simulink model "tqdtqr_rebuild_V3"  (R2021b)
settings: Solver=VariableStepAuto  StartTime=0.0  StopTime=10.0  RelTol=1e-3
undefined symbols (not defined in the file): ATQD_AfterTqMinGain_X_Deg, ATQD_APSCreepBaseTqD_X_kph, ATQD_APSCreepBaseTqD_Y_Deg, ATQD_APSCreepBaseTqR_X_kph, ATQD_APSCreepBaseTqR_Y_Deg, ATQD_APSCreepIterm_X_kph, ATQD_APSCreepIterm_Y_kph, ATQD_APSCreepPterm_X_kph, ATQD_APSCreepPterm_Y_kph, ATQD_APSDecReq_X_kph, ATQD_APSDecReq_Y_mps2, ATQD_APSDecReqCMD_X_kph, ATQD_APSDecReqTs_X_pct, ATQD_APSDecTimeGain_X_Deg, ATQD_APSDecTimeGain_Y_s, ATQD_APSReqLowSpd_X_Deg, ATQD_AutoHoldReleaseBPS_X_Deg, ATQD_AWDLoadTrqnsGain_X_kg, ATQD_AWDLoadTrqnsGain_Y_pct, ATQD_BOSEnBPSPosn_X_kph, ATQD_BOSMap_X_rpm, ATQD_BOSMap_Y_pct, ATQD_CreepBaseTqD_X_kph, ATQD_CreepBaseTqD_Y_Deg, ATQD_CreepBaseTqR_X_kph, ATQD_CreepBaseTqR_Y_Deg, ATQD_CreepBPSDisPosn_X_Deg, ATQD_CreepBPSDisPosnR_X_Deg, ATQD_CreepBPSEnPosn_X_Deg, ATQD_CreepBPSEnPosnR_X_Deg, ATQD_CreepDeltaTq_X_kph, ATQD_CreepIterm_X_kph, ATQD_CreepIterm_Y_kph, ATQD_CreepItermMaxLimit_X_pct, ATQD_CreepPreloadTime_X_kph, ATQD_CreepPreloadTq_X_kph, ATQD_CreepPreloadTq_Y_s, ATQD_CreepProtTq_X_Deg, ATQD_CreepPterm_X_kph, ATQD_CreepPterm_Y_kph, ATQD_CreepRrTqSpRat_X_rpm, ATQD_CreepRrTqSpRat_Y_Nm, ATQD_CreepTargetSpdD_X_pct, ATQD_CreepTargetSpdR_X_pct, ATQD_CreepUpLimitTq_X_rpm, ATQD_DecIneOPDHoldEnDelay_X_Deg, ATQD_DecIneOPDHoldEnDelay_Y_bar, ATQD_ECOTqMapD_X_rpm, ATQD_ECOTqMapD_Y_pct, ATQD_EMTqMapD_X_rpm, ATQD_EMTqMapD_Y_pct, ATQD_EOPDTqMapDCon_X_rpm, ATQD_EOPDTqMapDCon_Y_Deg, ATQD_EstInitVehWeight_X_c, ATQD_FAfterTqCMDGain_X_rpm, ATQD_FAfterTqCMDGain_Y_pct, ATQD_ForceLowSpd_X_Deg, ATQD_ForcePLimitSpd_X_Deg, ATQD_FrLossMAPLowV_X_rpm, ATQD_FrLossMAPLowV_Y_Nm ... (+949)
libraries: simulink x235, hcu_lib x208, tqr x63, tqd x6
(part 13 of 37)

== system tqdtqr_rebuild_V3/Input_Convert/Signal function/SWC1 SWC2 status ==
  note: SWC1 SWC2 result merge
  note: SWC2 status
  note: SWC1 status
  BSCPIn_outputs : Inport
  BSignalConvert_outputs : Inport  Port=2
  VTQD_GearActualPosn_enum : Inport  Port=3
  Bus Selector : BusSelector  OutputSignals=task_time_s,VINP_SWCResUpSta_flg,VINP_SWCSetdownSta_flg,VINP_SWCACCSta_flg,VINP_SWCCANCELSta_flg,VINP_IVIISAOffsetSpd_enum,VINP_ADASISASta_enum,VPMM_PowerSta_enum,VINP_ADASACCSta_enum,VVMC_CCCtrlSta_enum,VVMC_MSACtrlSta_enum,VINP_ADASVehSpdLim_enum,VVMC_LVDAACCStatusInformation_flg,VVMC_ACCObjDist_m,VVMC_MeterIndSpeed_raw32,VINP_Distanceunit_flg,VINP_SmartEcoModeSW_flg,VVMC_SetACCDisableAPS_flg,VINP_SWC2LScrollUpSta_flg,VINP_SWC2LScrollDownSta_flg,VINP_SWC2LScrollPressSta_flg,VINP_SWC2LADASSta_flg,VVMC_ADASActive_flg,VVMC_MSAActive_flg,VINP_ADASSLIFSpdLim_enum,VINP_IVIACCAdaptiveSta_flg,VTQD_LowIdleAccPedal_flg,VINP_SWCType_enum
  Bus Selector1 : BusSelector  OutputSignals=VTQD_ShiftGearPosn_enum
  Constant{1..3,90} (4 alike) : Constant  Value=ENUM_SWCTYPE_SWC2
  Constant77 : Constant  Value=ENUM_SWCTYPE_SWC
  Constant{78,82,84,89} (4 alike) : Constant  Value=FALSE
  Data Type Conversion4 : DataTypeConversion  OutDataTypeStr=boolean
  Data Type Conversion5 : DataTypeConversion  OutDataTypeStr=boolean
  Equal{1..3,30,40} (5 alike) : RelationalOperator  Operator===  OutDataTypeStr=boolean  RndMeth=Simplest
  SWC2_Subsystem : Subsystem  TreatAsAtomicUnit=on
  SWC_Subsystem : Subsystem
  Switch : Switch  Criteria=u2 ~= 0
      settings: AttributesFormatString=%<Criteria>
  Switch1 : Switch  Criteria=u2 ~= 0
      settings: AttributesFormatString=%<Criteria>
  Switch2 : Switch  Criteria=u2 ~= 0
      settings: AttributesFormatString=%<Criteria>
  VTQD_SWCResUpSta_flg : Outport
  VTQD_SWCSetdownSta_flg : Outport  Port=2
  VTQD_SWCCancelSta_flg : Outport  Port=3
  VTQD_SpdCtrlMode_enum : Outport  Port=4
  VTQD_SpdCtrlSta_flg : Outport  Port=5
  VTQD_SetSpd_kph : Outport  Port=6
  VTQD_SWC2ResUpSta_flg : Outport  Port=7
  VTQD_SWC2SetdownSta_flg : Outport  Port=8
  VTQD_SWC2CancelSta_flg : Outport  Port=9
  VTQD_SWC2LADASSta_flg : Outport  Port=10
  VTQD_SpdLim4SetSpd_raw32 : Outport  Port=11
  VTQD_SWC2ScrollUpSta_flg : Outport  Port=12
  VTQD_SWC1SetSpd_kph : Outport  Port=13
  VTQD_SWC2SetSpd_kph : Outport  Port=14
  wires:
  [VVMC_CCCtrlSta_enum] -> SWC_Subsystem/14(VVMC_CCCtrlSta_enum)
  [VINP_ADASACCSta_enum] -> SWC_Subsystem/11(VINP_ADASACCSta_enum)
  [VPMM_PowerSta_enum] -> SWC_Subsystem/10(VPMM_PowerSta_enum)
  [VINP_SWCACCSta_flg] -> SWC_Subsystem/6(VINP_SWCACCSta_flg)
  [VINP_SWCCANCELSta_flg] -> SWC_Subsystem/8(VINP_SWCCANCELSta_flg)
  [VINP_IVIISAOffsetSpd_enum] -> SWC_Subsystem/9(VTQD_IVIISAOffsetSpd_enum)
  [VINP_ADASVehSpdLim_enum] -> SWC_Subsystem/16(VINP_ADASVehSpdLim_kph)
  [VVMC_ACCObjDist_m] -> SWC_Subsystem/19(VVMC_ACCObjDist_m)
  [VDDM_SWCACCSta_flg] -> SWC_Subsystem/5(VDDM_SWCACCSta_flg)
  SWC_Subsystem/4(VTQD_SWCSpdCtrlMode_enum) -> [VTQD_SWCSpdCtrlMode_enum]
  SWC_Subsystem/2(VTQD_SWCSetdownSta_flg) -> [VTQD_SWCSetdownSta_flg]
  [VDDM_SWCCANCELSta_flg] -> SWC_Subsystem/7(VDDM_SWCCANCELSta_flg)
  Constant77/1 -> Equal30/2
  SWC_Subsystem/1(VTQD_SWCResUpSta_flg) -> [VTQD_SWCResUpSta_flg]
  [VDDM_SWCResUpSta_flg] -> SWC_Subsystem/1(VDDM_SWCResUpSta_flg)
  SWC_Subsystem/5(VTQD_SWCSpdCtrlSta_flg) -> [VTQD_SWCSpdCtrlSta_flg]
  Equal30/1 -> Data Type Conversion4/1
  Constant78/1 -> [VDDM_SWCResUpSta_flg]  "VDDM_SWCRegenUpSta_flg"
  SWC_Subsystem/6(VTQD_SWC1SetSpd_kph) -> [VTQD_SWC1SetSpd_kph]
  [VVMC_MeterIndSpeed_raw32] -> SWC_Subsystem/20(VVMC_MeterIndSpeed_raw32)
  [VINP_ADASISASta_enum] -> SWC_Subsystem/12(VINP_ADASISASta_enum)
  Constant82/1 -> [VDDM_SWCSetdownSta_flg]  "VDDM_SWCRegenDownSta_flg"
  Constant84/1 -> [VDDM_SWCACCSta_flg]  "VDDM_SWCRegenDownSta_flg"
  [VINP_SWCResUpSta_flg] -> SWC_Subsystem/2(VINP_SWCResUpSta_flg)
  Data Type Conversion4/1 -> SWC_Subsystem/Enable
  [VDDM_SWCSetdownSta_flg] -> SWC_Subsystem/3(VDDM_SWCSetdownSta_flg)
  [VTQD_ShiftGearPosn_enum] -> SWC_Subsystem/13(VTQD_ShiftGearPosn_enum)
  [VVMC_LVDAACCStatusInformation_flg] -> SWC_Subsystem/18(VVMC_LVDAACCStatusInformation_flg)
  [VINP_SWCSetdownSta_flg] -> SWC_Subsystem/4(VINP_SWCSetdownSta_flg)
  Constant89/1 -> [VDDM_SWCCANCELSta_flg]  "VDDM_SWCRegenDownSta_flg"
  [task_time_s] -> SWC_Subsystem/17(task_time_s)
  [VVMC_SetACCDisableAPS_flg] -> SWC_Subsystem/23(VVMC_SetACCDisableAPS_flg)
  [VINP_Distanceunit_flg] -> SWC_Subsystem/21(VINP_Distanceunit_flg)
  [VINP_SmartEcoModeSW_flg] -> SWC_Subsystem/22(VINP_SmartEcoModeSW_flg)
  [VVMC_MSACtrlSta_enum] -> SWC_Subsystem/15(VVMC_MSACtrlSta_enum)
  [VINP_SWCType_enum] -> Equal30/1
  SWC_Subsystem/3(VTQD_SWCCancelSta_flg) -> [VTQD_SWCCancelSta_flg]
  BSCPIn_outputs/1 -> Bus Selector/1
  Bus Selector/2 -> [VINP_SWCResUpSta_flg]  "<VINP_SWCResUpSta_flg>"
  Bus Selector/3 -> [VINP_SWCSetdownSta_flg]  "<VINP_SWCSetdownSta_flg>"
  Bus Selector/4 -> [VINP_SWCACCSta_flg]  "<VINP_SWCACCSta_flg>"
  Bus Selector/5 -> [VINP_SWCCANCELSta_flg]  "<VINP_SWCCANCELSta_flg>"
  Bus Selector/6 -> [VINP_IVIISAOffsetSpd_enum]  "<VINP_IVIISAOffsetSpd_enum>"
  Bus Selector/7 -> [VINP_ADASISASta_enum]  "<VINP_ADASISASta_enum>"
  Bus Selector/8 -> [VPMM_PowerSta_enum]  "<VPMM_PowerSta_enum>"
  Bus Selector/9 -> [VINP_ADASACCSta_enum]  "<VINP_ADASACCSta_enum>"
  Bus Selector/1 -> [task_time_s]  "<task_time_s>"
  Bus Selector/15 -> [VVMC_MeterIndSpeed_raw32]  "<VVMC_MeterIndSpeed_raw32>"
  Bus Selector/17 -> [VINP_SmartEcoModeSW_flg]  "<VINP_SmartEcoModeSW_flg>"
  Bus Selector/18 -> [VVMC_SetACCDisableAPS_flg]  "<VVMC_SetACCDisableAPS_flg>"
  Bus Selector/19 -> [VINP_SWC2LScrollUpSta_flg]  "<VINP_SWC2LScrollUpSta_flg>"
  Bus Selector/20 -> [VINP_SWC2LScrollDownSta_flg]  "<VINP_SWC2LScrollDownSta_flg>"
  Bus Selector/24 -> [VVMC_MSAActive_flg]  "<VVMC_MSAActive_flg>"
  Bus Selector/26 -> [VINP_IVIACCAdaptiveSta_flg]  "<VINP_IVIACCAdaptiveSta_flg>"
  Bus Selector/25 -> [VINP_ADASSLIFSpdLim_enum]  "<VINP_ADASSLIFSpdLim_enum>"
  Bus Selector/27 -> [VTQD_LowIdleAccPedal_flg]  "<VTQD_LowIdleAccPedal_flg>"
  VTQD_GearActualPosn_enum/1 -> [VTQD_GearActualPosn_enum]
  BSignalConvert_outputs/1 -> Bus Selector1/1
  Bus Selector1/1 -> [VTQD_ShiftGearPosn_enum]  "<VTQD_ShiftGearPosn_enum>"
  Bus Selector/28 -> [VINP_SWCType_enum]  "<VINP_SWCType_enum>"
  Bus Selector/10 -> [VVMC_CCCtrlSta_enum]  "<VVMC_CCCtrlSta_enum>"
  Bus Selector/11 -> [VVMC_MSACtrlSta_enum]  "<VVMC_MSACtrlSta_enum>"
  Bus Selector/12 -> [VINP_ADASVehSpdLim_enum]  "<VINP_ADASVehSpdLim_enum>"
  Bus Selector/13 -> [VVMC_LVDAACCStatusInformation_flg]  "<VVMC_LVDAACCStatusInformation_flg>"
  Bus Selector/14 -> [VVMC_ACCObjDist_m]  "<VVMC_ACCObjDist_m>"
  Bus Selector/16 -> [VINP_Distanceunit_flg]  "<VINP_Distanceunit_flg>"
  Bus Selector/21 -> [VINP_SWC2LScrollPressSta_flg]  "<VINP_SWC2LScrollPressSta_flg>"
  Bus Selector/22 -> [VINP_SWC2LADASSta_flg]  "<VINP_SWC2LADASSta_flg>"
  Bus Selector/23 -> [VVMC_ADASActive_flg]  "<VVMC_ADASActive_flg>"
  [VINP_SWC2LScrollUpSta_flg] -> SWC2_Subsystem/1(VINP_SWC2LScrollUpSta_flg)
  Data Type Conversion5/1 -> SWC2_Subsystem/Enable
  [VINP_SWC2LScrollDownSta_flg] -> SWC2_Subsystem/2(VINP_SWC2LScrollDownSta_flg)
  [VINP_Distanceunit_flg] -> SWC2_Subsystem/17(VINP_Distanceunit_flg)
  Equal40/1 -> Data Type Conversion5/1
  Constant90/1 -> Equal40/2
  [VVMC_MSAActive_flg] -> SWC2_Subsystem/8(VVMC_MSAActive_flg)
  [VVMC_CCCtrlSta_enum] -> SWC2_Subsystem/19(VVMC_CCCtrlSta_enum)
  SWC2_Subsystem/2(VTQD_SWC2SetdownSta_flg) -> [VTQD_SWC2SetdownSta_flg]
  [VINP_SWC2LADASSta_flg] -> SWC2_Subsystem/4(VINP_SWC2LADASSta_flg)
  [VTQD_GearActualPosn_enum] -> SWC2_Subsystem/5(VTQD_GearActualPosn_enum)
  [VTQD_ShiftGearPosn_enum] -> SWC2_Subsystem/15(VTQD_ShiftGearPosn_enum)
  [VPMM_PowerSta_enum] -> SWC2_Subsystem/14(VPMM_PowerSta_enum)
  [VINP_ADASACCSta_enum] -> SWC2_Subsystem/9(VINP_ADASACCSta_enum)
  SWC2_Subsystem/4(VTQD_SWC2LADASSta_flg) -> [VTQD_SWC2LADASSta_flg]
  [VINP_SWC2LScrollPressSta_flg] -> SWC2_Subsystem/3(VINP_SWC2LScrollPressSta_flg)
  [VINP_IVIACCAdaptiveSta_flg] -> SWC2_Subsystem/18(VINP_IVIACCAdaptiveSta_flg)
  SWC2_Subsystem/3(VTQD_SWC2CancelSta_flg) -> [VTQD_SWC2CancelSta_flg]  "VTQD_SWC2CancelSta_flg"
  [VVMC_ADASActive_flg] -> SWC2_Subsystem/6(VVMC_ADASActive_flg)
  [task_time_s] -> SWC2_Subsystem/12(task_time_s)
  [VINP_SmartEcoModeSW_flg] -> SWC2_Subsystem/20(VINP_SmartEcoModeSW_flg)
  [VINP_IVIISAOffsetSpd_enum] -> SWC2_Subsystem/13(VINP_IVIISAOffsetSpd_enum)
  SWC2_Subsystem/1(VTQD_SWC2ResUpSta_flg) -> [VTQD_SWC2ResUpSta_flg]
  [VVMC_MSACtrlSta_enum] -> SWC2_Subsystem/16(VVMC_MSACtrlSta_enum)
  [VINP_ADASSLIFSpdLim_enum] -> SWC2_Subsystem/11(VINP_ADASSLIFSpdLim_enum)
  SWC2_Subsystem/7(VTQD_SWC2SpdCtrlSta_flg) -> [VTQD_SWC2SpdCtrlSta_flg]
  [VINP_SWCType_enum] -> Equal40/1
  SWC2_Subsystem/6(VTQD_SpdCtrlMode_enum) -> [VTQD_SWC2SpdCtrlMode_enum]
  SWC2_Subsystem/5(VTQD_SpdLim4SetSpd_raw32) -> [VTQD_SpdLim4SetSpd_raw32]
  [VVMC_MeterIndSpeed_raw32] -> SWC2_Subsystem/10(VVMC_MeterIndSpeed_raw32)
  [VVMC_LVDAACCStatusInformation_flg] -> SWC2_Subsystem/7(VVMC_LVDAACCStaInfor_flg)
  [VTQD_LowIdleAccPedal_flg] -> SWC2_Subsystem/21(VTQD_LowIdleAccPedal_flg)
  [VTQD_SWCResUpSta_flg] -> VTQD_SWCResUpSta_flg/1
  [VTQD_SWCSetdownSta_flg] -> VTQD_SWCSetdownSta_flg/1
  [VTQD_SWCCancelSta_flg] -> VTQD_SWCCancelSta_flg/1
  [VTQD_SpdCtrlMode_enum] -> VTQD_SpdCtrlMode_enum/1
  [VTQD_SetSpd_kph] -> VTQD_SetSpd_kph/1
  [VTQD_SWC2ResUpSta_flg] -> VTQD_SWC2ResUpSta_flg/1
  [VTQD_SWC2SetdownSta_flg] -> VTQD_SWC2SetdownSta_flg/1
  [VTQD_SWC2CancelSta_flg] -> VTQD_SWC2CancelSta_flg/1
  [VTQD_SWC2LADASSta_flg] -> VTQD_SWC2LADASSta_flg/1
  [VTQD_SpdLim4SetSpd_raw32] -> VTQD_SpdLim4SetSpd_raw32/1
  SWC2_Subsystem/9(VTQD_SWC2ScrollUpSta_flg) -> [VTQD_SWC2ScrollUpSta_flg]
  [VTQD_SWC2ScrollUpSta_flg] -> VTQD_SWC2ScrollUpSta_flg/1
  [VTQD_SpdCtrlSta_flg] -> VTQD_SpdCtrlSta_flg/1
  SWC2_Subsystem/8(VTQD_SWC2SetSpd_kph) -> [VTQD_SWC2SetSpd_kph]
  [VINP_SWCType_enum] -> Equal1/1
  Constant1/1 -> Equal1/2
  Equal1/1 -> Switch/2
  [VTQD_SWC1SetSpd_kph] -> Switch/1
  [VTQD_SWC2SetSpd_kph] -> Switch/3
  Switch/1 -> [VTQD_SetSpd_kph]  "VTQD_SetSpd_kph"
  [VTQD_SWC1SetSpd_kph] -> VTQD_SWC1SetSpd_kph/1
  [VTQD_SWC2SetSpd_kph] -> VTQD_SWC2SetSpd_kph/1
  [VINP_SWCType_enum] -> Equal2/1
  Equal2/1 -> Switch1/2
  Constant2/1 -> Equal2/2
  Switch1/1 -> [VTQD_SpdCtrlMode_enum]  "VTQD_SpdCtrlMode_enum"
  [VTQD_SWC2SpdCtrlMode_enum] -> Switch1/3
  [VTQD_SWCSpdCtrlMode_enum] -> Switch1/1
  [VINP_SWCType_enum] -> Equal3/1
  Equal3/1 -> Switch2/2
  Constant3/1 -> Equal3/2
  [VTQD_SWC2SpdCtrlSta_flg] -> Switch2/3
  [VTQD_SWCSpdCtrlSta_flg] -> Switch2/1
  Switch2/1 -> [VTQD_SpdCtrlSta_flg]  "VTQD_SpdCtrlSta_flg"

== system tqdtqr_rebuild_V3/Input_Convert/Signal function/ShiftModule ==
  BSCPIn_outputs : Inport
  BSignalConvert_outputs : Inport  Port=2
  VTQD_EPBCarWashMode_flg : Inport  Port=3
  SWC_RegenUp : Inport  Port=4
  SWC_RegenDown : Inport  Port=5
  DriverWhlTqDemFunc_outputs : Inport  Port=6
  BMain_outputs : Inport  Port=7
  VTQD_OPDHoldAllowPark_flg : Inport  Port=8
  Bus Selector : BusSelector  OutputSignals=task_time_s,VPMM_PowerSta_enum,VINP_DrDoorSW_flg,VVMC_APSShiftPosnReq_enum,VVMC_APSActive_flg,VINP_DriverSeatBeltCmd_flg,VINP_ChrgPlugSta_enum,VINP_DOASta_flg,VINP_CAASSta_enum,VDDM_VCURAPSErrLv2_flg,VDDM_VCURAPSErrLv3_flg,VINP_APSStaSystem_enum,VDDM_Shifter1Err_flg,VDDM_ShifterSigErrCFS_flg,VTQD_ShifterHandleCmd_enum,VTQD_ShifterFailsta_enum,VINP_VehSpeed_kph,VINP_EPBSta_enum,VVMC_EstSlope_Deg,VPMM_DrSeatSta_enum,VTQD_ShifterHandleCmd_enum
  Bus Selector1 : BusSelector  OutputSignals=VTQD_BrkSwSta_flg,VTQD_VehActSpd_kph,VTQD_TMRotateDirction_enum,VTQD_IVIPwrLock_flg,VTQD_FrShaftSpd_rpm,VTQD_RrShaftSpd_rpm
  Bus Selector2 : BusSelector  OutputSignals=VTQD_IVIRockModeEn_flg
  Bus Selector3 : BusSelector  OutputSignals=VTQD_AfterAvailableTqDemFr_Nm,VTQD_AfterAvailableTqDemRr_Nm,VTQR_NoABSFEDUWhlTqReq_Nm,VTQR_NoABSREDUWhlTqReq_Nm
  Constant6 : Constant  Value=ENUM_GEARACTUALPOSN_P
  Constant7 : Constant  Value=ENUM_GEARACTUALPOSN_P
  Data Type Conversion1 : DataTypeConversion
  Data Type Conversion2 : DataTypeConversion
  Data Type Conversion3 : DataTypeConversion  OutDataTypeStr=uint8
  Data Type Conversion4 : DataTypeConversion  OutDataTypeStr=boolean
  Determin Gear State Configuration : Subsystem
  Determine_Actual_Gear_Position : Stateflow chart  TreatAsAtomicUnit=on
  Equal : RelationalOperator  Operator===  OutDataTypeStr=boolean  RndMeth=Simplest
  Equal1 : RelationalOperator  Operator=~=  OutDataTypeStr=boolean  RndMeth=Simplest
  Gear Shift Posn Cmd : Subsystem  Description=GearPosition
  SR_Latch : hcu_lib/Basic_Blocks/SR_Latch
  SR_Latch1 : Subsystem  mask(SR_Latch){}
      mask help: SR latch function.
  VTQD_GearActualPosn_enum : Outport
  VTQD_ParkRequest_flg : Outport  Port=2
  VTQD_PBWLockTO_flg : Outport  Port=3
  VTQD_PBWUnlockTO_flg : Outport  Port=4
  VTQD_DriveProtRemove_flg : Outport  Port=5
  VTQD_DriveProtEn_flg : Outport  Port=6
  VTQD_ForceP_flg : Outport  Port=7
  VTQD_DOALatchReq_flg : Outport  Port=8
  VTQD_ForcePLimitSpd_kph : Outport  Port=9
  wires:
  BSCPIn_outputs/1 -> Bus Selector/1
  Bus Selector/1 -> [task_time_s]  "<task_time_s>"
  Bus Selector/2 -> [VPMM_PowerSta_enum]  "<VPMM_PowerSta_enum>"
  Bus Selector/3 -> [VINP_DrDoorSW_flg]  "<VINP_DrDoorSW_flg>"
  Bus Selector/4 -> [VVMC_APSShiftPosnReq_enum]  "<VVMC_APSShiftPosnReq_enum>"
  Bus Selector/5 -> [VVMC_APSActive_flg]  "<VVMC_APSActive_flg>"
  Bus Selector/6 -> [VINP_DriverSeatBeltCmd_flg]  "<VINP_DriverSeatBeltCmd_flg>"
  Bus Selector/7 -> [VINP_ChrgPlugSta_enum]  "<VINP_ChrgPlugSta_enum>"
  Bus Selector/8 -> [VINP_DOASta_flg]  "<VINP_DOASta_flg>"
  Bus Selector/9 -> [VINP_CAASSta_enum]  "<VINP_CAASSta_enum>"
  Bus Selector/10 -> [VDDM_VCURAPSErrLv2_flg]  "<VDDM_VCURAPSErrLv2_flg>"
  Bus Selector/14 -> [VDDM_ShifterSigErrCFS_flg]  "<VDDM_ShifterSigErrCFS_flg>"
  Bus Selector/13 -> [VDDM_Shifter1Err_flg]  "<VDDM_Shifter1Err_flg>"
  Bus Selector/12 -> [VINP_APSStaSystem_enum]  "<VINP_APSStaSystem_enum>"
  Bus Selector/11 -> [VDDM_VCURAPSErrLv3_flg]  "<VDDM_VCURAPSErrLv3_flg>"
  BSignalConvert_outputs/1 -> Bus Selector1/1
  Bus Selector1/1 -> [VTQD_BrkSwSta_flg]  "<VTQD_BrkSwSta_flg>"
  Bus Selector1/3 -> [VTQD_TMRotateDirction_enum]  "<VTQD_TMRotateDirction_enum>"
  Bus Selector1/4 -> [VTQD_IVIPwrLock_flg]  "<VTQD_IVIPwrLock_flg>"
  Bus Selector1/5 -> [VTQD_FrShaftSpd_rpm]  "<VTQD_FrShaftSpd_rpm>"
  Bus Selector1/6 -> [VTQD_RrShaftSpd_rpm]  "<VTQD_RrShaftSpd_rpm>"
  [VTQD_GearActualPosn_enum] -> VTQD_GearActualPosn_enum/1
  [VTQD_DriveProtRemove_flg] -> VTQD_DriveProtRemove_flg/1
  [VTQD_DriveProtEn_flg] -> VTQD_DriveProtEn_flg/1
  [VTQD_ForceP_flg] -> VTQD_ForceP_flg/1
  [VTQD_PBWUnlockTO_flg] -> VTQD_PBWUnlockTO_flg/1
  [VTQD_PBWLockTO_flg] -> VTQD_PBWLockTO_flg/1
  [VTQD_ParkRequest_flg] -> VTQD_ParkRequest_flg/1
  SWC_RegenDown/1 -> [SWC_RegenDown]
  SWC_RegenUp/1 -> [SWC_RegenUp]
  VTQD_EPBCarWashMode_flg/1 -> [VTQD_EPBCarWashMode_flg]
  Bus Selector/15 -> [VTQD_ShifterHandleCmd_enum]  "<VTQD_ShifterHandleCmd_enum>"
  Bus Selector/16 -> [VTQD_ShifterFailsta_enum]  "<VTQD_ShifterFailsta_enum>"
  Determine_Actual_Gear_Position/3(VTQD_PBWUnlockTO_flg) -> Data Type Conversion2/1
  Data Type Conversion2/1 -> SR_Latch1/1(set)
  Data Type Conversion3/1 -> [VTQD_GearActualPosn_enum]  "VTQD_GearActualPosn_enum"
  Constant7/1 -> Equal1/2
  Determine_Actual_Gear_Position/4(VTQD_ParkRequest_flg) -> Data Type Conversion4/1
  [VTQD_GearActualPosn_enum] -> Equal1/1
  [VTQD_ShifterHandleCmd_enum] -> Gear Shift Posn Cmd/1(VTQD_ShifterHandleCmd_enum)
  [VINP_DriverSeatBeltCmd_flg] -> Gear Shift Posn Cmd/6(VINP_DriverSeatBeltCmd_flg)
  Gear Shift Posn Cmd/3(VTQD_PwrStaAllowDR_flg) -> [VTQD_PwrStaAllowDR_flg]
  Gear Shift Posn Cmd/2(VTQD_PwrStaAllowPN_flg) -> [VTQD_PwrStaAllowPN_flg]
  [VINP_APSStaSystem_enum] -> Gear Shift Posn Cmd/23(VINP_APSStaSystem_enum)
  Constant6/1 -> Equal/2
  Equal/1 -> SR_Latch/2
  [VTQD_OPDHoldAllowPark_flg] -> Gear Shift Posn Cmd/19(VTQD_OPDHoldAllowPark_flg)
  [VTQD_ShifterFailsta_enum] -> Gear Shift Posn Cmd/28(VTQD_ShifterFailsta_enum)
  SR_Latch1/1(latched) -> [VTQD_PBWUnlockTO_flg]  "VTQD_PBWUnlockTO_flg"
  [VDDM_Shifter1Err_flg] -> Gear Shift Posn Cmd/24(VDDM_Shifter1Err_flg)
  [VDDM_VCURAPSErrLv3_flg] -> Gear Shift Posn Cmd/22(VDDM_VCURAPSErrLv3_flg)
  [VTQD_GearActualPosn_enum] -> Equal/1
  [VPMM_PowerSta_enum] -> Gear Shift Posn Cmd/2(VPMM_PowerSta_enum)
  [VTQD_AfterAvailableTqDemFr_Nm] -> Gear Shift Posn Cmd/11(VTQD_AfterAvailableTqDemFr_Nm)
  [SWC_RegenDown] -> Gear Shift Posn Cmd/26(SWC_RegenDown)
  Determine_Actual_Gear_Position/1(VTQD_GearActualPosn_enum) -> Data Type Conversion3/1
  Data Type Conversion4/1 -> [VTQD_ParkRequest_flg]  "VTQD_ParkRequest_flg"
  [task_time_s] -> Gear Shift Posn Cmd/15(task_time_s)
  [VINP_DrDoorSW_flg] -> Gear Shift Posn Cmd/3(VINP_DrDoorSW_flg)
  Data Type Conversion1/1 -> SR_Latch/1
  [VINP_CAASSta_enum] -> Gear Shift Posn Cmd/20(VINP_CAASSta_enum)
  [VDDM_VCURAPSErrLv2_flg] -> Gear Shift Posn Cmd/21(VDDM_VCURAPSErrLv2_flg)
  [VTQD_BrkSwSta_flg] -> Gear Shift Posn Cmd/18(VTQD_BrkSwSta_flg)
  [VTQD_EPBCarWashMode_flg] -> Gear Shift Posn Cmd/7(VTQD_EPBCarWashMode_flg)
  [VINP_DOASta_flg] -> Gear Shift Posn Cmd/16(VINP_DOASta_flg)
  [VTQD_IVIPwrLock_flg] -> Gear Shift Posn Cmd/17(VTQD_IVIPwrLock_flg)
  Gear Shift Posn Cmd/1(VTQD_GearShiftCMD_enum) -> [VTQD_GearShiftCMD_enum]
  Gear Shift Posn Cmd/6(VTQD_ForceP_flg) -> [VTQD_ForceP_flg]
  [VINP_ChrgPlugSta_enum] -> Gear Shift Posn Cmd/9(VINP_ChrgPlugSta_enum)
  [VTQR_NoABSREDUWhlTqReq_Nm] -> Gear Shift Posn Cmd/14(VTQR_NoABSREDUWhlTqReq_Nm)
  Determine_Actual_Gear_Position/2(VTQD_PBWLockTO_flg) -> Data Type Conversion1/1
  [VDDM_ShifterSigErrCFS_flg] -> Gear Shift Posn Cmd/27(VDDM_ShifterSigErrCFS_flg)
  [VTQD_AfterAvailableTqDemRr_Nm] -> Gear Shift Posn Cmd/12(VTQD_AfterAvailableTqDemRr_Nm)
  Equal1/1 -> SR_Latch1/2(reset)
  [VVMC_APSShiftPosnReq_enum] -> Gear Shift Posn Cmd/4(VVMC_APSShiftPosnReq_enum)
  [VTQD_GearActualPosn_enum] -> Gear Shift Posn Cmd/10(VTQD_GearActualPosn_enum)
  [VTQR_NoABSFEDUWhlTqReq_Nm] -> Gear Shift Posn Cmd/13(VTQR_NoABSFEDUWhlTqReq_Nm)
  [VVMC_APSActive_flg] -> Gear Shift Posn Cmd/5(VVMC_APSActive_flg)
  [SWC_RegenUp] -> Gear Shift Posn Cmd/25(SWC_RegenUp)
  Gear Shift Posn Cmd/4(VTQD_DriveProtRemove_flg) -> [VTQD_DriveProtRemove_flg]
  Gear Shift Posn Cmd/5(VTQD_DriveProtEn_flg) -> [VTQD_DriveProtEn_flg]
  SR_Latch/1 -> [VTQD_PBWLockTO_flg]  "VTQD_PBWLockTO_flg"
  [VTQD_BrkSwSta_flg] -> Determin Gear State Configuration/1(VTQD_BrkSwSta_flg)
  [VTQD_GearShiftCMD_enum] -> Determin Gear State Configuration/2(VTQD_GearShiftCMD_enum)
  [VINP_VehSpeed_kph] -> Determin Gear State Configuration/3(VINP_VehSpeed_kph)
  [VTQD_PwrStaAllowDR_flg] -> Determin Gear State Configuration/4(VTQD_PwrStaAllowDR_flg)
  [VTQD_PwrStaAllowPN_flg] -> Determin Gear State Configuration/5(VTQD_PwrStaAllowPN_flg)
  [VTQD_TMRotateDirction_enum] -> Determin Gear State Configuration/6(VTQD_TMRotateDirction_enum)
  [VTQD_EPBCarWashMode_flg] -> Determin Gear State Configuration/7(VTQD_EPBCarWashMode_flg)
  [VVMC_APSActive_flg] -> Determin Gear State Configuration/8(VVMC_APSActive_flg)
  [VTQD_ForceP_flg] -> Determin Gear State Configuration/9(VTQD_ForceP_flg)
  [VTQD_IVIRockModeEn_flg] -> Determin Gear State Configuration/10(VTQD_IVIRockModeEn_flg)
  [VTQD_MaxShaftSpd_rpm] -> Determin Gear State Configuration/11(VTQD_MaxShaftSpd_rpm)
  Determin Gear State Configuration/1(VTQD_GearP2N_flg) -> [VTQD_GearP2N_flg]
  Determin Gear State Configuration/2(VTQD_GearN2P_flg) -> [VTQD_GearN2P_flg]
  Determin Gear State Configuration/3(VTQD_GearP2D_flg) -> [VTQD_GearP2D_flg]
  Determin Gear State Configuration/4(VTQD_GearD2P_flg) -> [VTQD_GearD2P_flg]
  Determin Gear State Configuration/5(VTQD_GearP2R_flg) -> [VTQD_GearP2R_flg]
  Determin Gear State Configuration/6(VTQD_GearR2P_flg) -> [VTQD_GearR2P_flg]
  Determin Gear State Configuration/7(VTQD_GearN2D_flg) -> [VTQD_GearN2D_flg]
  Determin Gear State Configuration/8(VTQD_GearD2N_flg) -> [VTQD_GearD2N_flg]
  Determin Gear State Configuration/9(VTQD_GearD2R_flg) -> [VTQD_GearD2R_flg]
  Determin Gear State Configuration/10(VTQD_GearR2D_flg) -> [VTQD_GearR2D_flg]
  Determin Gear State Configuration/11(VTQD_GearN2R_flg) -> [VTQD_GearN2R_flg]
  Determin Gear State Configuration/12(VTQD_GearR2N_flg) -> [VTQD_GearR2N_flg]
  [VTQD_GearP2N_flg] -> Determine_Actual_Gear_Position/2(VTQD_GearP2N_flg)
  [VTQD_GearN2P_flg] -> Determine_Actual_Gear_Position/3(VTQD_GearN2P_flg)
  [VTQD_GearP2D_flg] -> Determine_Actual_Gear_Position/4(VTQD_GearP2D_flg)
  [VTQD_GearD2P_flg] -> Determine_Actual_Gear_Position/5(VTQD_GearD2P_flg)
  [VTQD_GearP2R_flg] -> Determine_Actual_Gear_Position/6(VTQD_GearP2R_flg)
  [VTQD_GearR2P_flg] -> Determine_Actual_Gear_Position/7(VTQD_GearR2P_flg)
  [VTQD_GearN2D_flg] -> Determine_Actual_Gear_Position/8(VTQD_GearN2D_flg)
  [VTQD_GearD2N_flg] -> Determine_Actual_Gear_Position/9(VTQD_GearD2N_flg)
  [VTQD_GearD2R_flg] -> Determine_Actual_Gear_Position/10(VTQD_GearD2R_flg)
  [VTQD_GearR2D_flg] -> Determine_Actual_Gear_Position/11(VTQD_GearR2D_flg)
  [VTQD_GearN2R_flg] -> Determine_Actual_Gear_Position/12(VTQD_GearN2R_flg)
  [VTQD_GearR2N_flg] -> Determine_Actual_Gear_Position/13(VTQD_GearR2N_flg)
  Determine_Actual_Gear_Position/5(VTQD_ExitP_flg) -> [VTQD_ExitP_flg]
  Determine_Actual_Gear_Position/6(VTQD_EnterP_flg) -> [VTQD_EnterP_flg]
  [VTQD_ExitP_flg] -> Determin Gear State Configuration/12(VTQD_ExitP_flg)
  [VTQD_EnterP_flg] -> Determin Gear State Configuration/13(VTQD_EnterP_flg)
  [VTQD_FrShaftSpd_rpm] -> Gear Shift Posn Cmd/29(VTQD_FrShaftSpd_rpm)
  [VTQD_RrShaftSpd_rpm] -> Gear Shift Posn Cmd/30(VTQD_RrShaftSpd_rpm)
  Gear Shift Posn Cmd/7(VTQD_MaxShaftSpd_rpm) -> [VTQD_MaxShaftSpd_rpm]
  [task_time_s] -> Determine_Actual_Gear_Position/1(task_time_s)
  DriverWhlTqDemFunc_outputs/1 -> Bus Selector2/1
  Bus Selector2/1 -> [VTQD_IVIRockModeEn_flg]  "<VTQD_IVIRockModeEn_flg>"
  BMain_outputs/1 -> Bus Selector3/1
  Bus Selector3/1 -> [VTQD_AfterAvailableTqDemFr_Nm]  "<VTQD_AfterAvailableTqDemFr_Nm>"
  Bus Selector3/2 -> [VTQD_AfterAvailableTqDemRr_Nm]  "<VTQD_AfterAvailableTqDemRr_Nm>"
  Bus Selector3/3 -> [VTQR_NoABSFEDUWhlTqReq_Nm]  "<VTQR_NoABSFEDUWhlTqReq_Nm>"
  Bus Selector3/4 -> [VTQR_NoABSREDUWhlTqReq_Nm]  "<VTQR_NoABSREDUWhlTqReq_Nm>"
  VTQD_OPDHoldAllowPark_flg/1 -> [VTQD_OPDHoldAllowPark_flg]
  Bus Selector1/2 -> [VTQD_VehActSpd_kph]  "<VTQD_VehActSpd_kph>"
  Bus Selector/17 -> [VINP_VehSpeed_kph]  "<VINP_VehSpeed_kph>"
  [VTQD_VehActSpd_kph] -> Gear Shift Posn Cmd/8(VTQD_VehActSpd_kph)
  [VINP_EPBSta_enum] -> Gear Shift Posn Cmd/31(VINP_EPBSta_enum)
  Bus Selector/18 -> [VINP_EPBSta_enum]  "<VINP_EPBSta_enum>"
  [VINP_VehSpeed_kph] -> Gear Shift Posn Cmd/32(VINP_VehSpeed_kph)
  [VVMC_EstSlope_Deg] -> Gear Shift Posn Cmd/33(VVMC_EstSlope_Deg)
  Bus Selector/19 -> [VVMC_EstSlope_Deg]  "<VVMC_EstSlope_Deg>"
  [VPMM_DrSeatSta_enum] -> Gear Shift Posn Cmd/34(VPMM_DrSeatSta_enum)
  Bus Selector/20 -> [VPMM_DrSeatSta_enum]  "<VPMM_DrSeatSta_enum>"
  Gear Shift Posn Cmd/8(VTQD_DOALatchReq_flg) -> [VTQD_DOALatchReq_flg]
  Gear Shift Posn Cmd/9(VTQD_ForcePLimitSpd_kph) -> [VTQD_ForcePLimitSpd_kph]
  [VTQD_DOALatchReq_flg] -> VTQD_DOALatchReq_flg/1
  [VTQD_ForcePLimitSpd_kph] -> VTQD_ForcePLimitSpd_kph/1
  [VINP_ShifterHandleCmd_enum] -> Gear Shift Posn Cmd/35(VINP_ShifterHandleCmd_enum)
  Bus Selector/21 -> [VINP_ShifterHandleCmd_enum]  "<VTQD_ShifterHandleCmd_enum>"

== system tqdtqr_rebuild_V3/Input_Convert/Signal function/Simulation Sound Wave ==
  note: Simulation Sound Wave Command
  note: System Performance
  note: Simulation Sound Wave Request
  note: System Motor Power
  note: System Torque Power
  BSCPIn_outputs : Inport
  VTQD_GearActualPosn_enum : Inport  Port=2
  Abs : Abs
  Abs1 : Abs
  Add{,1..4} (5 alike) : Sum
  Bus Selector : BusSelector  OutputSignals=task_time_s,VINP_FrTMSpd_rpm,VINP_RrTMSpd_rpm,VINP_FrEDURealTMTq_Nm,VINP_RrEDURealTMTq_Nm,VTQD_ActAPSPosn_pct
  Constant : Constant  Value=PI
  Constant1 : Constant  Value=TWO_FLOAT
  Constant{3,5,10,15} (4 alike) : Constant  Value=EPS
  Constant11 : Constant  Value=KTQD_FrMotorRefPower_kW
  Constant12 : Constant  Value=ENUM_GEARACTUALPOSN_R
  Constant13 : Constant  Value=KTQD_FrUppTheldTrq_Nm
  Constant14 : Constant  Value=KTQD_RrUppTheldTrq_Nm
  Constant16 : Constant  Value=KTQD_SimSoundWaveSet_enum
  Constant17 : Constant  Value=ONE_INT
  Constant18 : Constant  Value=KTQD_SimSoundWaveSet_enum
  Constant19 : Constant  Value=TWO_INT
  Constant2 : Constant  Value=SIXTY
  Constant20 : Constant  Value=KTQD_SimSoundWaveSet_enum
  Constant21 : Constant  Value=THREE_INT
  Constant22 : Constant  Value=ZERO_FLOAT
  Constant23 : Constant  Value=KTQD_SimSoundWaveInc_pct
  Constant24 : Constant  Value=KTQD_SimSoundWaveDec_pct
  Constant4 : Constant  Value=KTQD_RrMotorRefPower_kW
  Constant6 : Constant  Value=THOUSAND
  Constant7 : Constant  Value=PI
  Constant8 : Constant  Value=TWO_FLOAT
  Constant9 : Constant  Value=SIXTY
  Data Type Conversion1 : DataTypeConversion  OutDataTypeStr=single
  Divide{,1..3} (4 alike) : Product  Inputs=*/
  Equal{,1..3} (4 alike) : RelationalOperator  Operator===  OutDataTypeStr=boolean  RndMeth=Simplest
  Gain : Gain  Gain=HUNDRED
  Gain2 : Gain  Gain=HUNDRED
  MINUSONE_FLOAT : Gain  Gain=MINUSONE_FLOAT
  Max{,1..3} (4 alike) : MinMax  Function=max  Inputs=2
  Product : Product  Inputs=4
  Product1 : Product
  Product2 : Product  Inputs=4
  RateLimit : hcu_lib/Basic_Blocks/RateLimit
  Relational Operator : RelationalOperator  OutDataTypeStr=boolean  RndMeth=Simplest
  Switch{,1..4} (5 alike) : Switch  Criteria=u2 ~= 0
      settings: AttributesFormatString=%<Criteria>
  VTQD_SimSouWaveReq_pct : Outport
  VTQD_SimSoundCmd_pct : Outport  Port=2
  wires:
  BSCPIn_outputs/1 -> Bus Selector/1
  Bus Selector/1 -> [task_time_s]  "<task_time_s>"
  Bus Selector/5 -> [VINP_RrEDURealTMTq_Nm]  "<VINP_RrEDURealTMTq_Nm>"
  Bus Selector/4 -> [VINP_FrEDURealTMTq_Nm]  "<VINP_FrEDURealTMTq_Nm>"
  Bus Selector/3 -> [VINP_RrTMSpd_rpm]  "<VINP_RrTMSpd_rpm>"
  Bus Selector/2 -> [VINP_FrTMSpd_rpm]  "<VINP_FrTMSpd_rpm>"
  VTQD_GearActualPosn_enum/1 -> [VTQD_GearActualPosn_enum]
  [VTQD_SimSouWaveReq_pct] -> VTQD_SimSouWaveReq_pct/1
  [VTQD_SimSoundCmd_pct] -> VTQD_SimSoundCmd_pct/1
  Bus Selector/6 -> [VTQD_ActAPSPosn_pct]  "<VTQD_ActAPSPosn_pct>"
  Constant1/1 -> Product/4
  [VTQD_ActAPSPosn_pct] -> Switch1/3
  [VINP_FrEDURealTMTq_Nm] -> Add2/1
  Constant16/1 -> Equal1/1
  [VTQD_SysMotorPower_pct] -> Switch2/1
  Add4/1 -> Max3/1
  [VTQD_SimSouWaveCMD_pct] -> RateLimit/1
  Product1/1 -> Max1/1
  Switch2/1 -> Switch3/3
  Switch4/1 -> [VTQD_SysMotorPerform_pct]  "VTQD_SysMotorPerform_pct"
  Constant11/1 -> Add/1
  Constant4/1 -> Add/2
  Add/1 -> Product1/1
  Constant22/1 -> RateLimit/2
  Gain2/1 -> [VTQD_SysMotorTorque_pct]  "VTQD_SysMotorTorque_pct"
  Constant17/1 -> Equal1/2
  Constant12/1 -> Equal/2
  [VINP_FrEDURealTMTq_Nm] -> Product/1
  Divide2/1 -> Gain/1
  Switch1/1 -> Switch2/3
  MINUSONE_FLOAT/1 -> Switch/1
  Constant7/1 -> Product2/3
  Constant18/1 -> Equal2/1
  Constant20/1 -> Equal3/1
  [VINP_RrTMSpd_rpm] -> Product2/2
  Max3/1 -> Divide3/2
  Constant23/1 -> RateLimit/4
  Add1/1 -> Divide2/1
  Constant19/1 -> Equal2/2
  Product2/1 -> Divide1/1
  Constant6/1 -> Product1/2
  [VINP_RrEDURealTMTq_Nm] -> Add2/2
  Switch3/1 -> [VTQD_SimSouWaveCMD_pct]  "VTQD_SimSouWaveCMD_pct"
  Equal/1 -> Switch/2
  Constant10/1 -> Max2/2
  Constant14/1 -> Add4/2
  Constant/1 -> Product/3
  Abs1/1 -> Relational Operator/2
  Max1/1 -> Divide2/2
  [VINP_FrEDURealTMTq_Nm] -> Add3/1
  Equal1/1 -> Switch1/2
  Max/1 -> Divide/2
  Divide1/1 -> [VTQD_RrMotorPwr_W]  "VTQD_RrMotorPwr_W"
  Constant9/1 -> Max2/1
  Constant8/1 -> Product2/4
  Add2/1 -> MINUSONE_FLOAT/1
  Relational Operator/1 -> Switch4/2
  Equal2/1 -> Switch2/2
  [VTQD_SysMotorPerform_pct] -> Switch3/1
  [VINP_RrEDURealTMTq_Nm] -> Product2/1
  [VTQD_RrMotorPwr_W] -> Add1/2
  Add3/1 -> Switch/3
  Abs/1 -> Relational Operator/1
  Gain/1 -> [VTQD_SysMotorPower_pct]  "VTQD_SysMotorPower_pct"
  Switch/1 -> Divide3/1
  RateLimit/1 -> [VTQD_SimSouWaveReq_pct], Data Type Conversion1/1  "VTQD_SimSouWaveReq_pct"
  [VTQD_SysMotorTorque_pct] -> Switch4/3
  [VTQD_SysMotorPower_pct] -> Switch4/1
  Constant3/1 -> Max/2
  [VTQD_GearActualPosn_enum] -> Equal/1
  Constant5/1 -> Max1/2
  Constant24/1 -> RateLimit/5
  Constant21/1 -> Equal3/2
  [VINP_FrTMSpd_rpm] -> Product/2
  Divide3/1 -> Gain2/1
  Product/1 -> Divide/1
  [VTQD_SysMotorTorque_pct] -> Switch1/1
  Constant15/1 -> Max3/2
  [VTQD_SysMotorPower_pct] -> Abs/1
  Constant2/1 -> Max/1
  Constant13/1 -> Add4/1
  [task_time_s] -> RateLimit/3
  [VTQD_FrMotorPwr_W] -> Add1/1
  Equal3/1 -> Switch3/2
  Max2/1 -> Divide1/2
  [VTQD_SysMotorTorque_pct] -> Abs1/1
  Divide/1 -> [VTQD_FrMotorPwr_W]  "VTQD_FrMotorPwr_W"
  [VINP_RrEDURealTMTq_Nm] -> Add3/2
  Data Type Conversion1/1 -> [VTQD_SimSoundCmd_pct]  "VTQD_SimSoundCmd_pct"

== system tqdtqr_rebuild_V3/Input_Convert/Signal function/VINP_EPBCarWashMode_flg ==
  BSCPIn_outputs : Inport
  AND1 : Logic  AllPortsSameDT=off  OutDataTypeStr=boolean
  AND2 : Logic  Inputs=4  AllPortsSameDT=off  OutDataTypeStr=boolean
  Bus Selector : BusSelector  OutputSignals=VINP_RollModeSWCmd_enum,VINP_DOASta_flg,VINP_EPBCarWashMode_flg,VINP_SCPSystemMode_enum,VINP_CAN2BusOff_flg,VINP_CAN2BusError_flg,VINP_CAN1BusOff_flg,VINP_CAN1BusError_flg,VDDM_EPB1NoComCFS_flg,VDDM_EPB1RCErrCFS_flg,VDDM_EPB1CSErrCFS_flg
  Constant1 : Constant  Value=ENUM_SYSMODE_MANUFACTURE
  Constant2 : Constant  Value=ENUM_ROLLMODESWCMD_PRESS
  Constant3 : Constant  Value=ENUM_ROLLMODESWCMD_RELEASE
  Delay1 : Delay  DelayLength=1  InitialCondition=boolean(0)
      settings: AttributesFormatString=%<InitialCondition>
  Equal1 : RelationalOperator  Operator===  OutDataTypeStr=boolean  RndMeth=Simplest
  Equal2 : RelationalOperator  Operator===  OutDataTypeStr=boolean  RndMeth=Simplest
  Equal3 : RelationalOperator  Operator===  OutDataTypeStr=boolean  RndMeth=Simplest
  NOT{1..2,5..6} (4 alike) : Logic  Operator=NOT  AllPortsSameDT=off  OutDataTypeStr=boolean
  OR1 : Logic  Operator=OR  Inputs=7  AllPortsSameDT=off  OutDataTypeStr=boolean
  OR7 : Logic  Operator=OR  AllPortsSameDT=off  OutDataTypeStr=boolean
  SR_Latch1 : hcu_lib/Basic_Blocks/SR_Latch
  Switch12 : Switch  Criteria=u2 ~= 0
      settings: AttributesFormatString=%<Criteria>
  Unit Delay1 : UnitDelay  InitialCondition=uint8(0)  SampleTime=-1  HasFrameUpgradeWarning=on
      settings: AttributesFormatString=%<InitialCondition>
  VTQD_EPBCarWashMode_flg : Outport
  wires:
  BSCPIn_outputs/1 -> Bus Selector/1
  Bus Selector/1 -> [VINP_RollModeSWCmd_enum]  "<VINP_RollModeSWCmd_enum>"
  Bus Selector/2 -> [VINP_DOASta_flg]  "<VINP_DOASta_flg>"
  Bus Selector/3 -> [VINP_EPBCarWashMode_flg]  "<VINP_EPBCarWashMode_flg>"
  [VTQD_EPBCarWashMode_flg] -> VTQD_EPBCarWashMode_flg/1
  [VDDM_EPB1CSErrCFS_flg] -> OR1/7
  Constant3/1 -> Equal3/2
  [VDDM_EPB1NoComCFS_flg] -> OR1/5
  [VINP_CAN1BusError_flg] -> OR1/4
  [VDDM_EPB1RCErrCFS_flg] -> OR1/6
  NOT5/1 -> AND2/3
  NOT2/1 -> OR7/2
  NOT1/1 -> OR1/2
  [VINP_EPBCarWashMode_flg] -> Switch12/3
  OR7/1 -> SR_Latch1/2
  [VINP_CAN2BusOff_flg] -> NOT5/1
  AND1/1 -> OR7/1
  SR_Latch1/1 -> Switch12/1
  OR1/1 -> NOT2/1, Switch12/2
  [VINP_CAN2BusError_flg] -> NOT6/1
  [VINP_CAN1BusOff_flg] -> OR1/3
  [VTQD_EPBCarWashMode_flg] -> Delay1/1
  [VINP_SCPSystemMode_enum] -> Equal1/1
  Constant2/1 -> Equal2/2
  [VINP_RollModeSWCmd_enum] -> Unit Delay1/1
  NOT6/1 -> AND2/4
  [VINP_RollModeSWCmd_enum] -> Equal3/1
  Equal1/1 -> OR1/1
  [VINP_DOASta_flg] -> NOT1/1
  Equal3/1 -> AND2/2
  Switch12/1 -> [VTQD_EPBCarWashMode_flg]  "VTQD_EPBCarWashMode_flg"
  Equal2/1 -> AND2/1
  Unit Delay1/1 -> Equal2/1
  Delay1/1 -> AND1/2
  AND2/1 -> SR_Latch1/1, AND1/1
  Constant1/1 -> Equal1/2
  Bus Selector/5 -> [VINP_CAN2BusOff_flg]  "<VINP_CAN2BusOff_flg>"
  Bus Selector/6 -> [VINP_CAN2BusError_flg]  "<VINP_CAN2BusError_flg>"
  Bus Selector/4 -> [VINP_SCPSystemMode_enum]  "<VINP_SCPSystemMode_enum>"
  Bus Selector/7 -> [VINP_CAN1BusOff_flg]  "<VINP_CAN1BusOff_flg>"
  Bus Selector/8 -> [VINP_CAN1BusError_flg]  "<VINP_CAN1BusError_flg>"
  Bus Selector/9 -> [VDDM_EPB1NoComCFS_flg]  "<VDDM_EPB1NoComCFS_flg>"
  Bus Selector/10 -> [VDDM_EPB1RCErrCFS_flg]  "<VDDM_EPB1RCErrCFS_flg>"
  Bus Selector/11 -> [VDDM_EPB1CSErrCFS_flg]  "<VDDM_EPB1CSErrCFS_flg>"

== system tqdtqr_rebuild_V3/Input_Convert/Signal function/VehWeightEst ==
  BSCPIn_outputs : Inport
  BSignalConvert_outputs : Inport  Port=2
  BMain_outputs : Inport  Port=3
  VTQD_GearActualPosn_enum : Inport  Port=4
  VTQD_FDCVCURegenMode_enum : Inport  Port=5
  Bus Selector : BusSelector  OutputSignals=task_time_s,VINP_VehSpeed_kph,VTQD_LowIdleAccPedal_flg,VINP_RrRBCActive_flg,VINP_FrRBCActive_flg,VINP_GRADE_Deg,VVMC_LongAcc_Gps,VINP_FrEDURealTMTq_Nm,VINP_RrEDURealTMTq_Nm,VINP_DriverSeatBeltCmd_flg,VINP_PsngrSeatBeltCmd_flg,VINP_RDriverSeatBeltCmd_flg,VINP_RCenterSeatBeltCmd_flg,VINP_RPsngrSeatBeltCmd_flg
  Bus Selector1 : BusSelector  OutputSignals=VTQD_RollRegenDisable_flg,VTQD_BrkSwSta_flg
  Bus Selector2 : BusSelector  OutputSignals=VTQD_AfterAvailableTqDemRr_Nm,VTQD_AfterAvailableTqDemFr_Nm,VTQR_NoABSREDUWhlTqReq_Nm,VTQR_NoABSFEDUWhlTqReq_Nm
  Calaulation : Subsystem
  Condition : Subsystem
  Desicion : Subsystem
  VTQD_EstVehWeightResult_kg : Outport
  wires:
  BSCPIn_outputs/1 -> Bus Selector/1
  Bus Selector/1 -> [task_time_s]  "<task_time_s>"
  Bus Selector/2 -> [VINP_VehSpeed_kph]  "<VINP_VehSpeed_kph>"
  Bus Selector/3 -> [VTQD_LowIdleAccPedal_flg]  "<VTQD_LowIdleAccPedal_flg>"
  Bus Selector/4 -> [VINP_RrRBCActive_flg]  "<VINP_RrRBCActive_flg>"
  Bus Selector/5 -> [VINP_FrRBCActive_flg]  "<VINP_FrRBCActive_flg>"
  Bus Selector/6 -> [VINP_GRADE_Deg]  "<VINP_GRADE_Deg>"
  Bus Selector/7 -> [VVMC_LongAcc_Gps]  "<VVMC_LongAcc_Gps>"
  Bus Selector/8 -> [VINP_FrEDURealTMTq_Nm]  "<VINP_FrEDURealTMTq_Nm>"
  Bus Selector/9 -> [VINP_RrEDURealTMTq_Nm]  "<VINP_RrEDURealTMTq_Nm>"
  Bus Selector/10 -> [VINP_DriverSeatBeltCmd_flg]  "<VINP_DriverSeatBeltCmd_flg>"
  Bus Selector/11 -> [VINP_PsngrSeatBeltCmd_flg]  "<VINP_PsngrSeatBeltCmd_flg>"
  Bus Selector/12 -> [VINP_RDriverSeatBeltCmd_flg]  "<VINP_RDriverSeatBeltCmd_flg>"
  Bus Selector/13 -> [VINP_RCenterSeatBeltCmd_flg]  "<VINP_RCenterSeatBeltCmd_flg>"
  Bus Selector/14 -> [VINP_RPsngrSeatBeltCmd_flg]  "<VINP_RPsngrSeatBeltCmd_flg>"
  BSignalConvert_outputs/1 -> Bus Selector1/1
  Bus Selector1/1 -> [VTQD_RollRegenDisableReq_flg]  "<VTQD_RollRegenDisable_flg>"
  Bus Selector1/2 -> [VTQD_BrkSwSta_flg]  "<VTQD_BrkSwSta_flg>"
  [VTQD_EstVehWeightResult_kg] -> VTQD_EstVehWeightResult_kg/1
  VTQD_GearActualPosn_enum/1 -> [VTQD_GearActualPosn_enum]
  VTQD_FDCVCURegenMode_enum/1 -> [VTQD_FDCVCURegenMode_enum]
  [VTQD_VehWeightEstEnd_flg] -> Condition/15(VTQD_VehWeightEstEnd_flg)
  [VINP_VehSpeed_kph] -> Calaulation/8(VINP_VehSpeed_kph)
  [VVMC_LongAcc_Gps] -> Calaulation/5(VVMC_LongAcc_Gps)
  [VINP_DriverSeatBeltCmd_flg] -> Desicion/4(VINP_DriverSeatBeltCmd_flg)
  [VTQD_VehWeightEstDis_flg] -> Desicion/2(VTQD_VehWeightEstDis_flg)
  [VINP_RPsngrSeatBeltCmd_flg] -> Desicion/8(VINP_RPsngrSeatBeltCmd_flg)
  [VTQD_EstVehWeight_kg] -> Desicion/3(VTQD_EstVehWeight_kg)
  [VTQD_EstRrRealTqCheckPass_flg] -> Desicion/11(VTQD_EstRrRealTqCheckPass_flg)
  [VTQD_EstFrRealTqCheckPass_flg] -> Desicion/10(VTQD_EstFrRealTqCheckPass_flg)
  [VINP_RDriverSeatBeltCmd_flg] -> Desicion/6(VINP_RDriverSeatBeltCmd_flg)
  Calaulation/3(VTQD_EstRrRealTqCheckPass_flg) -> [VTQD_EstRrRealTqCheckPass_flg]
  [VINP_FrEDURealTMTq_Nm] -> Calaulation/6(VINP_FrEDURealTMTq_Nm)
  Desicion/2(VTQD_EstVehWeightResult_kg) -> [VTQD_EstVehWeightResult_kg]
  [VINP_PsngrSeatBeltCmd_flg] -> Desicion/5(VINP_PsngrSeatBeltCmd_flg)
  [VTQD_AfterAvailableTqDemRr_Nm] -> Condition/1(VTQD_AfterAvailableTqDemRr_Nm)
  [VTQR_NoABSFEDUWhlTqReq_Nm] -> Condition/3(VTQR_NoABSFEDUWhlTqReq_Nm)
  [VINP_FrRBCActive_flg] -> Condition/12(VINP_FrRBCActive_flg)
  Condition/1(VTQD_VehWeightEstEn_flg) -> [VTQD_VehWeightEstEn_flg]
  [VINP_VehSpeed_kph] -> Condition/6(VINP_VehSpeed_kph)
  [VINP_RrEDURealTMTq_Nm] -> Calaulation/7(VINP_RrEDURealTMTq_Nm)
  [VTQD_LowIdleAccPedal_flg] -> Condition/9(VTQD_LowIdleAccPedal_flg)
  [VINP_GRADE_Deg] -> Condition/13(VINP_GRADE_Deg)
  [VTQD_AfterAvailableTqDemFr_Nm] -> Condition/4(VTQD_AfterAvailableTqDemFr_Nm)
  Desicion/1(VTQD_VehWeightEstEnd_flg) -> [VTQD_VehWeightEstEnd_flg]
  [VINP_RCenterSeatBeltCmd_flg] -> Desicion/7(VINP_RCenterSeatBeltCmd_flg)
  [task_time_s] -> Condition/14(task_time_s)
  Calaulation/1(VTQD_EstLongAccCheckPass_flg) -> [VTQD_EstLongAccCheckPass_flg]
  [VINP_RrRBCActive_flg] -> Condition/11(VINP_RrRBCActive_flg)
  [VTQD_EstLongAccCheckPass_flg] -> Desicion/9(VTQD_EstLongAccCheckPass_flg)
  [VTQD_FDCVCURegenMode_enum] -> Condition/8(VINP_RegenMode_enum)
  [task_time_s] -> Calaulation/1(task_time_s)
  [VTQD_VehWeightEstEn_flg] -> Calaulation/2(VTQD_VehWeightEstEn_flg)
  [VTQD_BrkSwSta_flg] -> Condition/10(VTQD_BrkSwSta_flg)
  [VTQD_GearActualPosn_enum] -> Condition/5(VTQD_GearActualPosn_enum)
  [VTQD_RollRegenDisableReq_flg] -> Condition/7(VTQD_RollRegenDisableReq_flg)
  Calaulation/2(VTQD_EstFrRealTqCheckPass_flg) -> [VTQD_EstFrRealTqCheckPass_flg]
  [VTQR_NoABSREDUWhlTqReq_Nm] -> Condition/2(VTQR_NoABSREDUWhlTqReq_Nm)
  Calaulation/4(VTQD_EstVehWeight_kg) -> [VTQD_EstVehWeight_kg]
  [VTQD_VehWeightEstDis_flg] -> Calaulation/3(VTQD_VehWeightEstDis_flg)
  Condition/2(VTQD_VehWeightEstDis_flg) -> [VTQD_VehWeightEstDis_flg]
  [VTQD_VehWeightEstEnd_flg] -> Calaulation/4(VTQD_VehWeightEstEnd_flg)
  [task_time_s] -> Desicion/1(task_time_s)
  BMain_outputs/1 -> Bus Selector2/1
  Bus Selector2/1 -> [VTQD_AfterAvailableTqDemRr_Nm]  "<VTQD_AfterAvailableTqDemRr_Nm>"
  Bus Selector2/2 -> [VTQD_AfterAvailableTqDemFr_Nm]  "<VTQD_AfterAvailableTqDemFr_Nm>"
  Bus Selector2/3 -> [VTQR_NoABSREDUWhlTqReq_Nm]  "<VTQR_NoABSREDUWhlTqReq_Nm>"
  Bus Selector2/4 -> [VTQR_NoABSFEDUWhlTqReq_Nm]  "<VTQR_NoABSFEDUWhlTqReq_Nm>"
